simulink library "lib_parallel_comp"  (Simulink 7.4)
settings: Solver=ode45  StartTime=0.0  StopTime=10.0  RelTol=1e-3
values from neighbouring files (symbols this model uses):
  n_delay = [0; 40]    [setup.m]
  P_D = x(end)    [comp_rig_parallel_linearized.m]    (also in comp_rig_tank.m = x(1); get_tank_deriv.m = x(1); setup.m = 0.9925; test_linearization.m = P_D_init + delta_x(end,i))
  Ts = 0.05    [const_sim.m]
  uoff1 = [0.304, 0.405, 0.393, 0]'    [const_sim.m]
  uoff2 = [0.304, 0.405, 0.393, 0]'    [const_sim.m]
  xinit = [0.898; 1.12; 0.152; 438; 0 ... (first row only)    [setup.m]    (also in test_linearization.m = [0.890; 1.096; 0.159; 426; 0)
libraries: lib_compressor x2
settings Model: Creator=chkajon  LastModifiedBy=chkajon

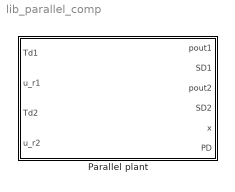
== system lib_parallel_comp ==
  Parallel plant : Subsystem  mask{x_init_total=xinit, disturbances_on=off, disturbances_symm=off, dist_t_in=0, dist1_in=0, dist2_in=0}
      mask prompts: x_init_total "Initial state"; disturbances_on "Activate disturbances"; disturbances_symm "Symmetric disturbances"; dist_t_in "Disturbance times (up to 2)"; dist1_in "Disturbance 1 values (u1in, u1out, ud[, u2in, u2out])"; dist2_in "Disturbance 2 values"
      mask init:
      | dist1 = zeros(5,1);
      | dist2 = dist1;
      | dist_t = zeros(2,1);
      | 
      | if disturbances_on
      |     for i=1:min(5,length(dist1_in))
      |         dist1(i) = dist1_in(i);
      |     end
      |     for i=1:min(5,length(dist2_in))
      |         dist2(i) = dist2_in(i);
      |     end
      |     for i=1:min(2,length(dist_t_in))
      |         dist_t(i) = dist_t_in(i);
      |     end
      |     
      |     if disturbances_symm
      |         dist1(4) = dist1(1);
      |         dist1(5) = dist1(2);
      |         dist2(4) = dist2(1);
      |         dist2(5) = dist2(2);
      |     end
      | end
      | 
      | x_init1 = x_init_total(1:5);
      | x_init2 = x_init_total(6:10);

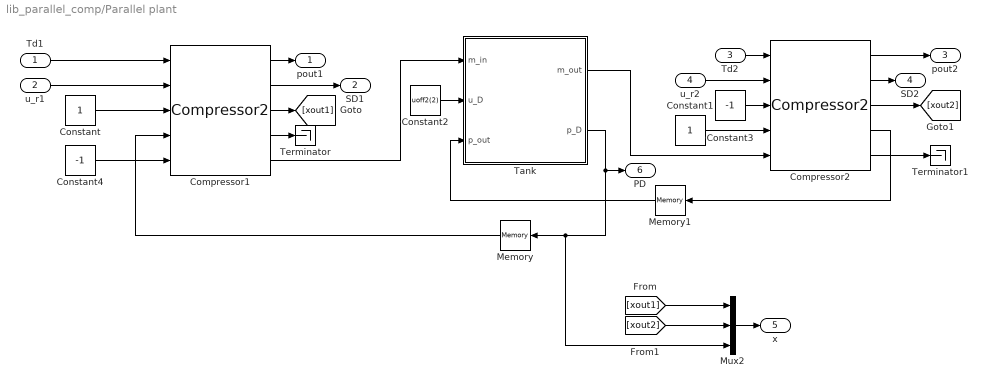
== system lib_parallel_comp/Parallel plant ==
  Td1 : Inport  OutDataType=fixdt(1, 16)  OutScaling=2^0
  u_r1 : Inport  Port=2  OutDataType=fixdt(1, 16)  OutScaling=2^0
  Td2 : Inport  Port=3  OutDataType=fixdt(1, 16)  OutScaling=2^0
  u_r2 : Inport  Port=4  OutDataType=fixdt(1, 16)  OutScaling=2^0
  Compressor1 : lib_compressor/Compressor2  SystemSampleTime=-1  x_init=x_init1  Td_off=uoff1(1)  u_in=uoff1(2)  u_out=uoff1(3)  u_rec=uoff1(4)  t_delay=n_delay(2)*Ts  use_dist=on  u_out_dist=[dist1(1); dist2(1)]  u_out_time=dist_t  u_in_dist=[dist1(2); dist2(2)]  u_in_time=dist_t
  Compressor2 : lib_compressor/Compressor2  SystemSampleTime=-1  x_init=x_init2  Td_off=uoff2(1)  u_in=uoff2(2)  u_out=uoff2(3)  u_rec=uoff2(4)  t_delay=n_delay(2)*Ts  use_dist=on  u_out_dist=[dist1(4); dist2(4)]  u_out_time=dist_t  u_in_dist=[dist1(5); dist2(5)]  u_in_time=dist_t
  Constant : Constant  OutDataType=fixdt(1, 16)  OutScaling=2^0
  Constant1 : Constant  OutDataType=fixdt(1, 16)  OutScaling=2^0
  Constant2 : Constant  Value=uoff2(2)  OutDataType=fixdt(1, 16)  OutScaling=2^0
  Constant3 : Constant  Value=-1  OutDataType=fixdt(1, 16)  OutScaling=2^0
  Constant4 : Constant  Value=-1  OutDataType=fixdt(1, 16)  OutScaling=2^0
  Memory : Memory  X0=P_D
  Memory1 : Memory  X0=x_init_total(6)
  Mux2 : Mux  Inputs=3
  Tank : Subsystem
  Terminator : Terminator
  Terminator1 : Terminator
  pout1 : Outport  OutDataType=fixdt(1, 16)  OutScaling=2^0
  SD1 : Outport  Port=2  OutDataType=fixdt(1, 16)  OutScaling=2^0
  pout2 : Outport  Port=3  OutDataType=fixdt(1, 16)  OutScaling=2^0
  SD2 : Outport  Port=4  OutDataType=fixdt(1, 16)  OutScaling=2^0
  x : Outport  Port=5  OutDataType=fixdt(1, 16)  OutScaling=2^0
  PD : Outport  Port=6  OutDataType=fixdt(1, 16)  OutScaling=2^0
  wires:
  Constant4/1 -> Compressor1/5
  Constant/1 -> Compressor1/3
  u_r1/1 -> Compressor1/2
  Td1/1 -> Compressor1/1
  Memory/1 -> Compressor1/4
  Compressor2/5 -> Terminator1/1
  Compressor1/4 -> Terminator/1
  Compressor1/5 -> Tank/1(m_in)
  Constant3/1 -> Compressor2/3
  Td2/1 -> Compressor2/1
  u_r2/1 -> Compressor2/2
  [xout1] -> Mux2/1
  [xout2] -> Mux2/2
  Mux2/1 -> x/1
  Compressor1/1 -> pout1/1
  Constant1/1 -> Compressor2/4
  Compressor1/2 -> SD1/1
  Compressor1/3 -> [xout1]
  Compressor2/1 -> pout2/1
  Compressor2/2 -> SD2/1
  Compressor2/3 -> [xout2]
  Tank/2(p_D) -> Mux2/3, Memory/1, PD/1
  Tank/1(m_out) -> Compressor2/5
  Constant2/1 -> Tank/2(u_D)
  Compressor2/4 -> Memory1/1
  Memory1/1 -> Tank/3(p_out)

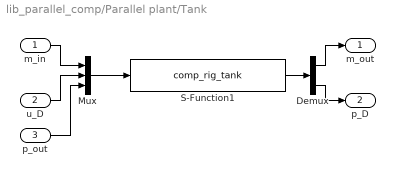
== system lib_parallel_comp/Parallel plant/Tank ==
  m_in : Inport  OutDataType=fixdt(1, 16)  OutScaling=2^0
  u_D : Inport  Port=2  OutDataType=fixdt(1, 16)  OutScaling=2^0
  p_out : Inport  Port=3  OutDataType=fixdt(1, 16)  OutScaling=2^0
  Demux : Demux  Outputs=2
  Mux : Mux  Inputs=3
  S-Function1 : S-Function  FunctionName=comp_rig_tank  Parameters=[], P_D  EnableBusSupport=off
  m_out : Outport  OutDataType=fixdt(1, 16)  OutScaling=2^0
  p_D : Outport  Port=2  OutDataType=fixdt(1, 16)  OutScaling=2^0
  wires:
  u_D/1 -> Mux/2
  m_in/1 -> Mux/1
  Mux/1 -> S-Function1/1
  Demux/2 -> p_D/1
  Demux/1 -> m_out/1
  S-Function1/1 -> Demux/1
  p_out/1 -> Mux/3
